simulink model "g1simulink"  (R2023b)
settings: Solver=VariableStepAuto  StartTime=0.0  StopTime=30  RelTol=1e-3
undefined symbols (not defined in the file): h1, h2
libraries: cstblocks x8
settings Model: Creator=klysm  LastModifiedBy=klysm

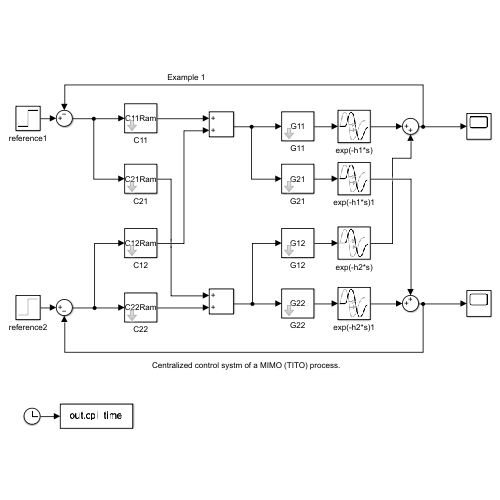
[thumbnail: Simulink's stored preview of the top-level diagram]
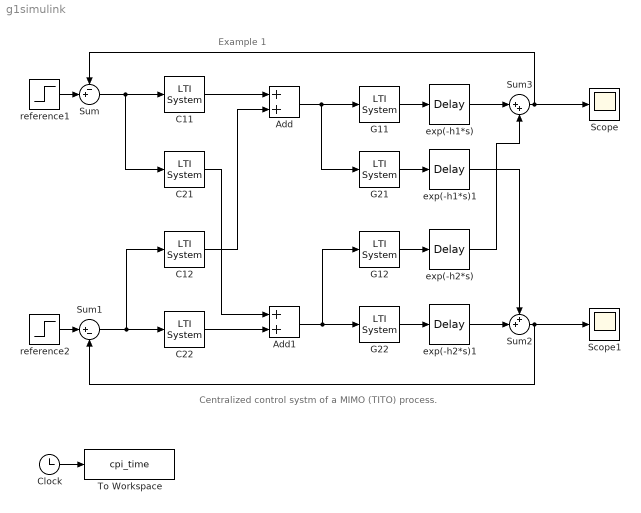
== system g1simulink ==
  note: Example 1
  note: Centralized control systm of a MIMO (TITO) process.
  Add : Sum
  Add1 : Sum
  C11 : cstblocks/LTI System  sys=C11Ram  IC=[]  PadeOrder=0
  C12 : cstblocks/LTI System  sys=C12Ram  IC=[]  PadeOrder=0
  C21 : cstblocks/LTI System  sys=C21Ram  IC=[]  PadeOrder=0
  C22 : cstblocks/LTI System  sys=C22Ram  IC=[]  PadeOrder=0
  Clock : Clock
  G11 : cstblocks/LTI System  sys=G11  IC=[]  PadeOrder=0
  G12 : cstblocks/LTI System  sys=G12  IC=[]  PadeOrder=0
  G21 : cstblocks/LTI System  sys=G21  IC=[]  PadeOrder=0
  G22 : cstblocks/LTI System  sys=G22  IC=[]  PadeOrder=0
  Scope : Scope
  Scope1 : Scope
  Sum : Sum  Inputs=-+|
  Sum1 : Sum  Inputs=|+-
  Sum2 : Sum  Inputs=++|
  Sum3 : Sum  Inputs=|++
  To Workspace : ToWorkspace  VariableName=cpi_time  SampleTime=-1
  exp(-h1*s) : TransportDelay  DelayTime=h1
  exp(-h1*s)1 : TransportDelay  DelayTime=h1
  exp(-h2*s) : TransportDelay  DelayTime=h2
  exp(-h2*s)1 : TransportDelay  DelayTime=h2
  reference1 : Step  Time=0  SampleTime=0
  reference2 : Step  Time=15  SampleTime=0
  wires:
  Clock/1 -> To Workspace/1
  reference2/1 -> Sum1/1
  reference1/1 -> Sum/2
  Sum/1 -> C21/1, C11/1
  Sum1/1 -> C12/1, C22/1
  C11/1 -> Add/1
  C12/1 -> Add/2
  C22/1 -> Add1/2
  C21/1 -> Add1/1
  Add/1 -> G21/1, G11/1
  Add1/1 -> G12/1, G22/1
  G22/1 -> exp(-h2*s)1/1
  G11/1 -> exp(-h1*s)/1
  G12/1 -> exp(-h2*s)/1
  G21/1 -> exp(-h1*s)1/1
  exp(-h2*s)1/1 -> Sum2/2
  exp(-h1*s)1/1 -> Sum2/1
  exp(-h1*s)/1 -> Sum3/1
  exp(-h2*s)/1 -> Sum3/2
  Sum2/1 -> Sum1/2, Scope1/1
  Sum3/1 -> Sum/1, Scope/1
